simulink model "SIMULINK_CONTROL_01"  (R2020a)
settings: Solver=FixedStepAuto  StartTime=0.0  StopTime=100  FixedStep=0.01  RelTol=1e-3
libraries: simulink x2
settings Model: Creator=alejandropuerta  LastModifiedBy=USUARIO

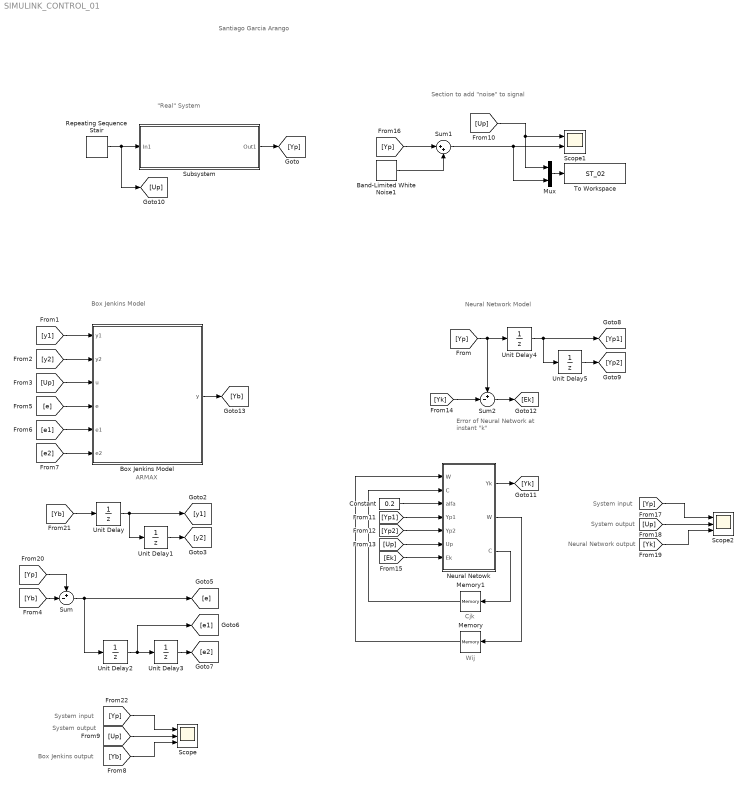
== system SIMULINK_CONTROL_01 ==
  note: Santiago Garcia Arango
  note: Wij
  note: Box Jenkins Model
  note: Error of Neural
      | Network at instant "k"
  note: ARMAX
  note: "Real" System
  note: Neural Network Model
  note: Cjk
  note: Section to add "noise" to signal
  note: System input
  note: System output
  note: Neural Network output
  note: Box Jenkins output
  note: System input
  note: System output
  Band-Limited White Noise1 : simulink/Sources/Band-Limited White Noise  Cov=[0.000001]  Ts=0.01  seed=[23341]
  Box Jenkins Model : MATLAB Function  TreatAsAtomicUnit=on
  Constant : Constant  Value=0.2
  Memory : Memory  InitialCondition=randn(10,3)
  Memory1 : Memory  InitialCondition=randn(1,10)
  Mux : Mux  Inputs=2
  Neural Netowk : MATLAB Function  TreatAsAtomicUnit=on
  Repeating Sequence Stair : simulink/Sources/Repeating Sequence Stair  OutValues=[0 0.2 0 0.4 0.8 0.4 1].'  tsamp=15  OutMin=[]  OutMax=[]  OutDataTypeStr=double  OutputDataTypeScalingMode=double  OutDataType=fixdt(0,8)  ConRadixGroup=Best Precision: Vector-wise  OutScaling=2^-12
  Scope : Scope  NumInputPorts=3
  Scope1 : Scope  NumInputPorts=2
  Scope2 : Scope  NumInputPorts=3
  Subsystem : Subsystem
  Sum : Sum  Inputs=+-|
  Sum1 : Sum  Inputs=|++
  Sum2 : Sum  Inputs=+-|
  To Workspace : ToWorkspace  VariableName=ST_02  SampleTime=-1
      settings: Save2DSignal=2-D array (concatenate along first dimension)
  Unit Delay{,1..5} (6 alike) : UnitDelay  SampleTime=-1  HasFrameUpgradeWarning=on
  wires:
  Subsystem/1(Out1) -> [Yp]
  Repeating Sequence Stair/1 -> [Up], Subsystem/1(In1)
  Box Jenkins Model/1(y) -> [Yb]
  Unit Delay/1 -> [y1], Unit Delay1/1
  Unit Delay1/1 -> [y2]
  [y1] -> Box Jenkins Model/1(y1)
  [y2] -> Box Jenkins Model/2(y2)
  [Up] -> Box Jenkins Model/3(u)
  [Yb] -> Sum/2
  Sum/1 -> Unit Delay2/1, [e]
  Unit Delay2/1 -> Unit Delay3/1, [e1]
  Unit Delay3/1 -> [e2]
  [e] -> Box Jenkins Model/4(e)
  [e1] -> Box Jenkins Model/5(e1)
  [e2] -> Box Jenkins Model/6(e2)
  [Yp] -> Sum1/1
  Sum1/1 -> Mux/2, Scope1/2
  [Up] -> Scope1/1, Mux/1
  Mux/1 -> To Workspace/1
  Unit Delay5/1 -> [Yp2]
  Unit Delay4/1 -> [Yp1], Unit Delay5/1
  [Yp] -> Sum2/1, Unit Delay4/1
  Constant/1 -> Neural Netowk/3(alfa)
  [Yp1] -> Neural Netowk/4(Yp1)
  [Yp2] -> Neural Netowk/5(Yp2)
  Neural Netowk/1(Yk) -> [Yk]
  [Yk] -> Sum2/2
  Sum2/1 -> [Ek]
  [Ek] -> Neural Netowk/7(Ek)
  [Up] -> Neural Netowk/6(Up)
  Neural Netowk/2(W) -> Memory/1
  Neural Netowk/3(C) -> Memory1/1
  Memory1/1 -> Neural Netowk/2("C ")
  Memory/1 -> Neural Netowk/1("W ")
  [Yp] -> Scope2/1
  [Up] -> Scope2/2
  [Yk] -> Scope2/3
  [Yp] -> Sum/1
  [Yb] -> Unit Delay/1
  [Up] -> Scope/2
  [Yp] -> Scope/1
  [Yb] -> Scope/3
  Band-Limited White Noise1/1 -> Sum1/2

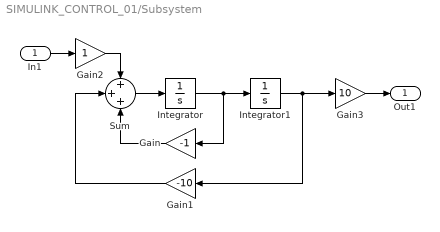
== system SIMULINK_CONTROL_01/Subsystem ==
  In1 : Inport
  Gain : Gain  Gain=-1
  Gain1 : Gain  Gain=-10
  Gain2 : Gain
  Gain3 : Gain  Gain=10
  Integrator : Integrator
  Integrator1 : Integrator
  Sum : Sum  Inputs=+++
  Out1 : Outport  VectorParamsAs1DForOutWhenUnconnected=off
  wires:
  Integrator/1 -> Integrator1/1, Gain/1
  Gain2/1 -> Sum/1
  Gain1/1 -> Sum/2
  Sum/1 -> Integrator/1
  Integrator1/1 -> Gain3/1, Gain1/1
  Gain/1 -> Sum/3
  In1/1 -> Gain2/1
  Gain3/1 -> Out1/1

== matlab function SIMULINK_CONTROL_01/Neural Netowk ==
  data: W input; Yk output; C input; alfa input; Yp1 input; Yp2 input; Up input; Ek input; W output; C output
% NEURAL NETWORK FOR SIMULINK "REAL-TIME" PROCESSING BASED ON SIGNALS
% Santiago Garcia Arango
% ------------------------------------------------------------------------
% FEEDFORWARDMADALINE. Train or Test a simple neural network.
%   alfa: Learning rate constant (1 x 1)
%   W: vector of the initial Weights. size (1 x ne)
%   C: matrix of the initial hidden layers weights. size (ns x no+1)
%   desired: matrix of the desired output, based on entries size (ns x nd)
%   activation_function_x: "none" to pass "Ys" directly.
%   Yp1, Yp2: Original system values (delays)
%   
% ------------------------------------------------------------------------

function [Yk, W, C] = fcn(W, C, alfa, Yp1, Yp2, Up, Ek)

activation_function_1 = "tanh";
activation_function_2 = "none";

X = [Yp1, Yp2, Up]; % Create "entries" vector
Aj = W*X'; % Add hidden layer

if (activation_function_1 == "tanh")
    H = tanh(Aj);
end

Ak = C'*H; % Add output layer

if (activation_function_2 == "none")
    Yk = Ak;
end

C = C+alfa*Ek*H; % Update weights of C

if (activation_function_1 == "tanh")
    H2 = sech(Aj).^2;
end

W = W+alfa*Ek*(C.*H2)*X; % Update weights of W

end

== matlab function SIMULINK_CONTROL_01/Box Jenkins Model ==
  data: y1 input; y2 input; u input; y output; e input; e1 input; e2 input
function y = fcn(y1,y2,u,e,e1,e2)

a1 = 1.989;
a2 = -0.99;
a3 = 0.0009799;
a4 = -1.967;
a5 = 0.9681;

y = a1*y1 + a2*y2 + a3*u + e + a4*e1 + a5*e2;
